simulink model "diagrama"  (R2026a)
settings: Solver=VariableStepAuto  StopTime=5  MaxStep=T/10
undefined symbols (not defined in the file or in its folder): dend, numd, T
settings Model: Creator=paludeto  LastModifiedBy=paludeto

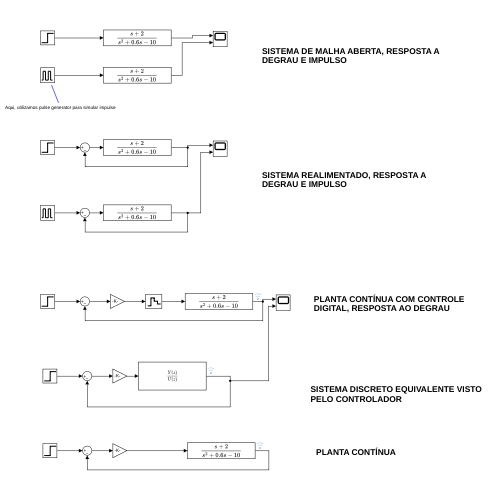
[thumbnail: Simulink's stored preview of the top-level diagram]
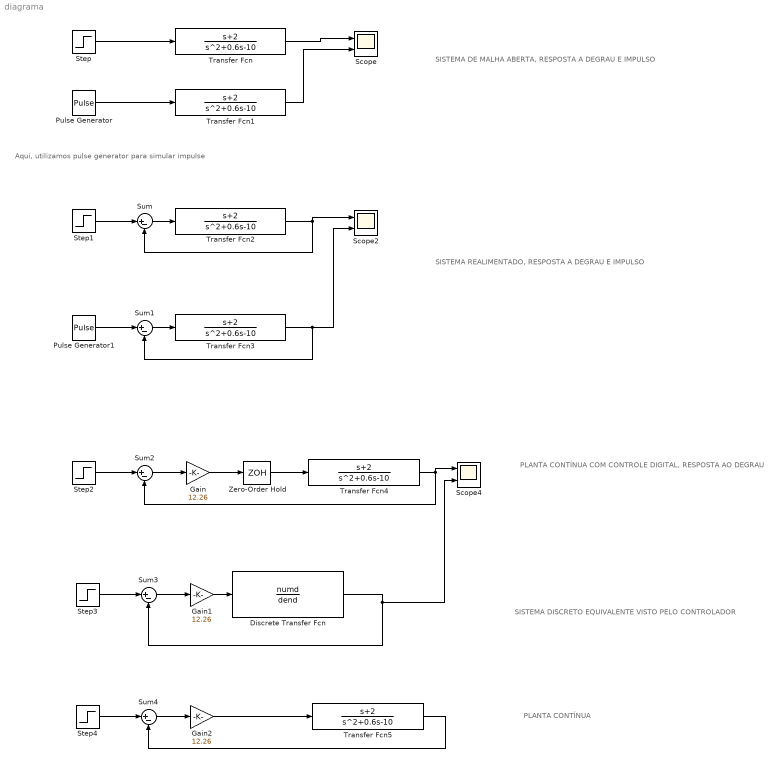
== system diagrama ==
  note: SISTEMA DE MALHA ABERTA, RESPOSTA A DEGRAU E IMPULSO
  note: Aqui, utilizamos pulse generator para simular impulse
  note: SISTEMA REALIMENTADO, RESPOSTA A DEGRAU E IMPULSO
  note: PLANTA CONTÍNUA COM CONTROLE DIGITAL, RESPOSTA AO DEGRAU
  note: SISTEMA DISCRETO EQUIVALENTE VISTO PELO CONTROLADOR
  note: PLANTA CONTÍNUA
  Discrete Transfer Fcn : DiscreteTransferFcn  Numerator=numd  Denominator=dend  SampleTime=T
  Gain : Gain  Gain=12.26
  Gain1 : Gain  Gain=12.26
  Gain2 : Gain  Gain=12.26
  Pulse Generator : DiscretePulseGenerator  PulseType=Time based  Amplitude=1000  Period=100  PulseWidth=0.001
  Pulse Generator1 : DiscretePulseGenerator  PulseType=Time based  Amplitude=1000  Period=100  PulseWidth=0.001
  Scope : Scope  NumInputPorts=2
      settings: ActiveDisplayYMinimum=-7260.6176828386251  ActiveDisplayYMaximum=65345.559145547639
  Scope2 : Scope  NumInputPorts=2
      settings: DataLoggingVariableName=ScopeData2
  Scope4 : Scope  NumInputPorts=2
      settings: DataLoggingVariableName=ScopeData4
  Step : Step  SampleTime=0
  Step1 : Step  SampleTime=0
  Step2 : Step  Time=0  SampleTime=0
  Step3 : Step  Time=0  SampleTime=0
  Step4 : Step  Time=0  SampleTime=0
  Sum{,1..4} (5 alike) : Sum  Inputs=|+-
  Transfer Fcn{,1..5} (6 alike) : TransferFcn  Numerator=[1 2]  Denominator=[1 0.6 -10]
  Zero-Order Hold : ZeroOrderHold  SampleTime=T
  wires:
  Step/1 -> Transfer Fcn/1
  Transfer Fcn/1 -> Scope/1
  Pulse Generator/1 -> Transfer Fcn1/1
  Transfer Fcn2/1 -> Sum/2, Scope2/1
  Step1/1 -> Sum/1
  Sum/1 -> Transfer Fcn2/1
  Pulse Generator1/1 -> Sum1/1
  Transfer Fcn3/1 -> Scope2/2, Sum1/2
  Sum1/1 -> Transfer Fcn3/1
  Step2/1 -> Sum2/1
  Sum2/1 -> Gain/1
  Gain/1 -> Zero-Order Hold/1
  Zero-Order Hold/1 -> Transfer Fcn4/1
  Transfer Fcn4/1 -> Sum2/2, Scope4/1
  Step3/1 -> Sum3/1
  Sum3/1 -> Gain1/1
  Gain1/1 -> Discrete Transfer Fcn/1
  Discrete Transfer Fcn/1 -> Scope4/2, Sum3/2
  Transfer Fcn1/1 -> Scope/2
  Step4/1 -> Sum4/1
  Transfer Fcn5/1 -> Sum4/2
  Sum4/1 -> Gain2/1
  Gain2/1 -> Transfer Fcn5/1
